simulink model "LKAS_AutoSave_20200911_1102"  (R2018b)
settings: Solver=FixedStepDiscrete  StartTime=0.0  StopTime=10.0  FixedStep=0.01  RelTol=1e-3
InitFcn:
  | tmpVer = ver('MATLAB');
  | tmpVer = str2num(tmpVer.Version);
  | % -------------------------------------------------------------------
  | %  MATLAB file generated by Simulink.saveVars on 21-Nov-2019 10:06:14
  | %  MATLAB version: 7.13.0.564 (R2011b)
  | % -------------------------------------------------------------------
  | 
  | 
  | SInt16 = Simulink.AliasType;
  | SInt16.Description = 'Num';
  | if (tmpVer > 7.11)
  | 	SInt16.DataScope = 'Auto';
  | end
  | SInt16.HeaderFile = 'Rte_Type.h';
  | SInt16.BaseType = 'int16';
  | 
  | SInt32 = Simulink.AliasType;
  | SInt32.Description = 'Num';
  | if (tmpVer > 7.11)
  | 	SInt32.DataScope = 'Auto';
  | end
  | SInt32.HeaderFile = 'Rte_Type.h';
  | SInt32.BaseType = 'int32';
  | 
  | SInt8 = Simulink.AliasType;
  | SInt8.Description = 'Num';
  | if (tmpVer > 7.11)
  | 	SInt8.DataScope = 'Auto';
  | end
  | SInt8.HeaderFile = 'Rte_Type.h';
  | SInt8.BaseType = 'int8';
  | 
  | T_A_m2_1024_1_u32 = Simulink.NumericType;
  | T_A_m2_1024_1_u32.Description = 'm2 (square meters  (m2))';
  | if (tmpVer > 7.11)
  | 	T_A_m2_1024_1_u32.DataScope = 'Auto';
  | end
  | T_A_m2_1024_1_u32.HeaderFile = 'Rte_Type.h';
  | T_A_m2_1024_1_u32.DataTypeMode = 'Fixed-point: slope and bias scaling';
  | T_A_m2_1024_1_u32.SignednessBool = false;
  | T_A_m2_1024_1_u32.WordLength = 32;
  | T_A_m2_1024_1_u32.FixedExponent = -10;
  | T_A_m2_1024_1_u32.SlopeAdjustmentFactor = 1;
  | T_A_m2_1024_1_u32.Bias = 0;
  | T_A_m2_1024_1_u32.DataTypeOverride = 'Inherit';
  | T_A_m2_1024_1_u32.IsAlias = true;
  | 
  | T_A_m2_65536_1_u16 = Simulink.NumericType;
  | T_A_m2_65536_1_u16.Description = 'm2 (square meters  (m2))';
  | if (tmpVer > 7.11)
  | 	T_A_m2_65536_1_u16.DataScope = 'Auto';
  | end
  | T_A_m2_65536_1_u16.HeaderFile = 'Rte_Type.h';
  | T_A_m2_65536_1_u16.DataTypeMode = 'Fixed-point: slope and bias scaling';
  | T_A_m2_65536_1_u16.SignednessBool = false;
  | T_A_m2_65536_1_u16.WordLength = 16;
  | T_A_m2_65536_1_u16.FixedExponent = -16;
  | T_A_m2_65536_1_u16.SlopeAdjustmentFactor = 1;
  | T_A_m2_65536_1_u16.Bias = 0;
  | T_A_m2_65536_1_u16.DataTypeOverride = 'Inherit';
  | ... (+4598 lines)
StopFcn:
  | clear  T_A_m2_1024_1_u32 T_A_m2_65536_1_u16 T_A_m2_Float32 T_A_mm2_10_1_u16 T_A_mm2_4_1_s16 T_A_mm2_Float32 T_Cnt_Num_10_1_u32 T_Cnt_Num_1_1_s16 T_Cnt_Num_1_1_s32 T_Cnt_Num_1_1_s8 T_Cnt_Num_1_1_u16 T_Cnt_Num_1_1_u32 T_Cnt_Num_1_1_u8 T_E_J_1_1_s32 T_E_J_Float32 T_E_kJ_128_1_s32 T_E_kJ_Float32 T_E_kwh_10_1_u16 T_E_kwh_Float32 T_Epl_kwhpkm_100_1_u16 T_Epl_kwhpkm_Float32 T_F_N_1_1_s16 T_F_N_Float32 T_I_A_1000_1_u16 T_I_A_1048576_1_s32 T_I_A_2048_1_s16 T_I_A_32_1_s16 T_I_A_Float32 T_I_mA_1_1_s16 T_I_mA_32768_128_s16 T_I_mA_Float32 T_J_kgpm2_128_1_u16 T_J_kgpm2_Float32 T_K_NA_1000_1_s16 T_K_NA_100_1_s16 T_K_NA_100_1_u16 T_K_NA_1024_1_s16 T_K_NA_1024_1_u16 T_K_NA_128_1_s16 T_K_NA_128_1_u16 T_K_NA_128_1_u8 T_K_NA_16777216_1_u32 T_K_NA_16_1_s16 T_K_NA_16_1_u16 T_K_NA_16_1_u8 T_K_NA_1_16_u16 T_K_NA_1_1_s16 T_K_NA_1_1_u16 T_K_NA_1_1_u8 T_K_NA_32768_1_s16 T_K_NA_32768_1_u16 T_K_NA_32_1_s8 T_K_NA_4096_1_u16 T_K_NA_4194304_1_s32 T_K_NA_4194304_1_u16 T_K_NA_65536_1_s32 T_K_NA_65536_1_u16 T_K_NA_8192_1_s16 T_K_NA_8_1_s16 T_K_NA_Float32 T_M_Nm_16_1_s16 T_M_Nm_1_1_s16 T_M_Nm_32768_1_s16 T_M_Nm_32_1_s16 T_M_Nm_4_1_s16 T_M_Nm_512_1_s16 T_M_Nm_Float32 T_P_W_1_4_s16 T_P_W_1_8_s16 T_P_W_Float32 T_P_kW_128_1_s16 T_P_kW_1_8_s16 T_P_kW_8_1_s32 T_P_kW_Float32 T_Pct_pct_1024_1_s32 T_Pct_pct_1024_1_u32 T_Pct_pct_10_1_s16 T_Pct_pct_10_1_u32 T_Pct_pct_128_100_s8 T_Pct_pct_1_1_s16 T_Pct_pct_1_4_u8 T_Pct_pct_255_100_u16 T_Pct_pct_255_100_u8 T_Pct_pct_256_1_s16 T_Pct_pct_256_1_u16 T_Pct_pct_65535_100_u16 T_Pct_pct_Float32 T_R_ohm_1024_1_s16 T_R_ohm_32_1_s16 T_R_ohm_Float32 T_TK_K_16_1_s16 T_TK_K_Float32 T_T_degC_10_400_1_u16 T_T_degC_16_1_s16 T_T_degC_1_40_1_u8 T_T_degC_2_80_1_u8 T_T_degC_Float32 T_U_V_1000_1_u16 T_U_V_10_1_u8 T_U_V_200_1_u8 T_U_V_32_1_s16 T_U_V_4096_1_s16 T_U_V_512_1_s16 T_U_V_65535_8_u16 T_U_V_8192_1_u16 T_U_V_Float32 T_U_mV_1_1_s16 T_U_mV_256_20_u16 T_U_mV_Float32 T_V_l_256_1_s16 T_V_l_4096_1_s16 T_V_l_64_1_s16 T_V_l_65535_100_u16 T_V_l_Float32 T_V_ml_128_1_s16 T_V_ml_1_1_s16 T_V_ml_32768_1_s16 T_V_ml_Float32 T_V_ul_32_1_u16 T_V_ul_Float32 T_Vpl_clpkm_512_1_u16 T_Vpl_clpkm_Float32 T_a_kphps_16_1_s16 T_a_kphps_Float32 T_a_mps2_128_1_s16 T_a_mps2_Float32 T_c_MJpkg_256_1_s16 T_c_MJpkg_Float32 T_c_kJpgpK_1024_1_s16 T_c_kJpgpK_Float32 T_c_kJpkgpK_128_1_u16 T_c_kJpkgpK_Float32 T_chrg_Ah_1_1_s16 T_chrg_Ah_1_1_u16 T_chrg_Ah_1_1_u8 T_chrg_Ah_256_1_u16 T_chrg_Ah_4194304_1_s32 T_chrg_Ah_512_1_u16 T_chrg_Ah_8_1_u16 T_chrg_Ah_Float32 T_cmp_NA_100_1_s16 T_cmp_NA_128_1_s16 T_cmp_NA_16_1_s16 T_cmp_NA_32768_1_u16 T_cmp_NA_Float32 T_d2n_rpmps2_4_1_s16 T_d2n_rpmps2_Float32 T_dPct_pctps_16_1_s16 T_dPct_pctps_256_1_s16 T_dPct_pctps_Float32 T_dT_degCps_128_1_s16 T_dT_degCps_Float32 T_dV_lph_1_1_s16 T_dV_lph_Float32 T_dV_lpm_128_1_s16 T_dV_lpm_32_1_s16 T_dV_lpm_Float32 T_dV_lps_1024_1_u16 T_dV_lps_4_1_u16 T_dV_lps_Float32 T_dV_mlps_1024_1_s16 T_dV_mlps_Float32 T_d_BitField16 T_dm_gps_128_1_s16 T_dm_gps_128_1_u16 T_dm_gps_256_1_u16 T_dm_gps_Float32 T_dm_mgps_1_1_s16 T_dm_mgps_Float32 T_dn_rpmps_1_1_s16 T_dn_rpmps_2_1_s16 T_dn_rpmps_Float32 T_dp_Paps_1_1_s16 T_dp_Paps_Float32 T_dp_kPaps_1_1_s16 T_dp_kPaps_8_1_s16 T_dp_kPaps_Float32 T_dphi_degps_128_1_s16 T_dphi_degps_8_1_s16 T_dphi_degps_Float32 T_dr_ps_256_1_s16 T_dr_ps_Float32 T_drho_mgplps_1_2_s16 T_drho_mgplps_Float32 T_e_NA_1_1_u8 T_f_Hz_1_1_u16 T_f_Hz_1_1_u32 T_f_Hz_64_1_u16 T_f_Hz_8_1_s16 T_f_Hz_Float32 T_g_BitField32 T_l_km_16_1_s16 T_l_km_1_1_u16 T_l_km_1_1_u32 T_l_km_Float32 T_l_m_1024_1_s16 T_l_m_16_1_s16 T_l_m_1_1_u32 T_l_m_Float32 T_l_mm_16_1_s16 T_l_mm_1_1_u16 T_l_mm_4096_1_s16 T_l_mm_4_1_u8 T_l_mm_64_1_s16 T_l_mm_Float32 T_m_g_1_1_s16 T_m_g_2048_1_s16 T_m_g_32_1_u16 T_m_g_Float32 T_m_kg_1024_1_s16 T_m_kg_1_1_s16 T_m_kg_1_1_u32 T_m_kg_Float32 T_m_mg_128_1_s16 T_m_mg_32_1_s16 T_m_mg_Float32 T_n_rpm_1_1_s16 T_n_rpm_1_25_u8 T_n_rpm_256_50_u16 T_n_rpm_2_25_u8 T_n_rpm_4_1_u16 T_n_rpm_Float32 T_p_MPa_64_1_s16 T_p_MPa_Float32 T_p_Pa_1_1_s16 T_p_Pa_Float32 T_p_kPa_1_10_u16 T_p_kPa_1_1_s16 T_p_kPa_1_1_u8 T_p_kPa_256_1_u16 T_p_kPa_32_1_u16 T_p_kPa_64_1_s16 T_p_kPa_Float32 T_phi_deg_100_1_s16 T_phi_deg_1024_1_s16 T_phi_deg_128_1_s16 T_phi_deg_1_1_u8 T_phi_deg_256_1_s16 T_phi_deg_2_1_s8 T_phi_deg_32_1_s16 T_phi_deg_512_6_s32 T_phi_deg_Float32 T_phi_rad_2048_1_s16 T_phi_rad_Float32 T_r_NA_1024_1_s16 T_r_NA_1024_1_u16 T_r_NA_16384_1_s16 T_r_NA_16_1_s16 T_r_NA_256_1_s8 T_r_NA_256_1_u16 T_r_NA_32768_1_u16 T_r_NA_32_1_u16 T_r_NA_4096_1_s16 T_r_NA_65535_2_u16 T_r_NA_8192_1_u16 T_r_NA_Float32 T_rho_gpl_8192_1_s16 T_rho_gpl_Float32 T_rho_kgpm3_16_1_s16 T_rho_kgpm3_Float32 T_rho_mgpl_1_1_s16 T_rho_mgpl_64_1_s16 T_rho_mgpl_Float32 T_t_hour_1_1_s16 T_t_hour_Float32 T_t_m_1_1_u16 T_t_m_Float32 T_t_ms_1_1_s16 T_t_ms_1_1_u16 T_t_ms_1_1_u32 T_t_ms_4096_1_s16 T_t_ms_64_1_s16 T_t_ms_Float32 T_t_s_1000_1_s16 T_t_s_100_1_s16 T_t_s_10_1_s16 T_t_s_10_1_u16 T_t_s_1_1_s16 T_t_s_1_1_u16 T_t_s_1_1_u32 T_t_s_Float32 T_t_us_10_1_u32 T_t_us_1_1_s16 T_t_us_1_1_u32 T_t_us_1_4_u16 T_t_us_Float32 T_v_kph_1_1_u8 T_v_kph_64_1_s16 T_v_kph_64_1_u16 T_v_kph_Float32 T_v_mps_256_1_s16 T_v_mps_Float32 T_w_radps_32_1_s16 T_w_radps_Float32 T_y_BitField8 T_y_BitFieldDiagProgress T_y_BitFieldDiagStatus T_y_NA_1_1_u8 SInt16 SInt32 SInt8 T_BOOLEAN UInt16 UInt32 UInt8 s16 s32 s8 u16 u32 u8
model workspace (MAT data in the model file):
  MCOS : class17 (value not decoded)
  MCOS : class17 (value not decoded)
  MCOS : class17 (value not decoded)
  MCOS : class17 (value not decoded)
  MCOS : class17 (value not decoded)
  MCOS : class17 (value not decoded)
  MCOS : class17 (value not decoded)
  MCOS : class17 (value not decoded)
  MCOS : class17 (value not decoded)
  MCOS : class17 (value not decoded)
  MCOS : class17 (value not decoded)
  MCOS : class17 (value not decoded)
  MCOS : class17 (value not decoded)
  MCOS : class17 (value not decoded)
  MCOS : class17 (value not decoded)
  MCOS : class17 (value not decoded)
  MCOS : class17 (value not decoded)
  MCOS : class17 (value not decoded)
  MCOS : class17 (value not decoded)
  MCOS : class17 (value not decoded)
  MCOS : class17 (value not decoded)
  MCOS : class17 (value not decoded)
  MCOS : class17 (value not decoded)
  MCOS : class17 (value not decoded)
  MCOS : class17 (value not decoded)
  MCOS : class17 (value not decoded)
  MCOS : class17 (value not decoded)
  MCOS : class17 (value not decoded)
  MCOS : class17 (value not decoded)
  MCOS : class17 (value not decoded)
  MCOS : class17 (value not decoded)
  MCOS : class17 (value not decoded)
  MCOS : class17 (value not decoded)
  MCOS : class17 (value not decoded)
  MCOS : class17 (value not decoded)
  MCOS : class17 (value not decoded)
  MCOS : class17 (value not decoded)
  MCOS : class17 (value not decoded)
  MCOS : class17 (value not decoded)
  MCOS : class17 (value not decoded)
  MCOS : class17 (value not decoded)
  MCOS : class17 (value not decoded)
  MCOS : class17 (value not decoded)
  MCOS : class17 (value not decoded)
  MCOS : class17 (value not decoded)
  MCOS : class17 (value not decoded)
  MCOS : class17 (value not decoded)
  MCOS : class17 (value not decoded)
  MCOS : class17 (value not decoded)
  MCOS : class17 (value not decoded)
  MCOS : class17 (value not decoded)
  MCOS : class17 (value not decoded)
  MCOS : class17 (value not decoded)
  MCOS : class17 (value not decoded)
  MCOS : class17 (value not decoded)
  MCOS : class17 (value not decoded)
  MCOS : class17 (value not decoded)
  MCOS : class17 (value not decoded)
  MCOS : class17 (value not decoded)
  MCOS : class17 (value not decoded)
  MCOS : class17 (value not decoded)
  MCOS : class17 (value not decoded)
  MCOS : class17 (value not decoded)
  MCOS : class17 (value not decoded)
  MCOS : class17 (value not decoded)
  MCOS : class17 (value not decoded)
  MCOS : class17 (value not decoded)
  MCOS : class17 (value not decoded)
  MCOS : class17 (value not decoded)
  MCOS : class17 (value not decoded)
  MCOS : class17 (value not decoded)
  MCOS : class17 (value not decoded)
  MCOS : class17 (value not decoded)
  MCOS : class17 (value not decoded)
  MCOS : class17 (value not decoded)
  MCOS : class17 (value not decoded)
  MCOS : class17 (value not decoded)
  MCOS : class17 (value not decoded)
  MCOS : class17 (value not decoded)
  MCOS : class17 (value not decoded)
  MCOS : class17 (value not decoded)
  MCOS : class17 (value not decoded)
  MCOS : class17 (value not decoded)
  MCOS : class17 (value not decoded)
  MCOS : class17 (value not decoded)
  MCOS : class17 (value not decoded)
  MCOS : class17 (value not decoded)
  MCOS : class17 (value not decoded)
  MCOS : class17 (value not decoded)
undefined symbols (not defined in the file): LKA_CarWidth, LKA_SampleTime, LKA_StrRatio_C, LKA_Veh2CamL_C, LKA_Veh2CamW_C, LKA_WhlBaseL_C, LL_CompSWA_C, LL_CrvtPrvwT_C, LL_DesDvt_C, LL_DvtComp_C, LL_DvtPrvwT_C, LL_DvtSpdDet_vDvtSpdMin_C, LL_HdAgExT_C, LL_HdAgPrvwT_C, LL_LAccMax_C, LL_LAccRMax_C, LL_LDW_EarliestWarnLine_C, LL_LDW_LatestWarnLine_C, LL_LDWS_SUPPRESS_HEADING, LL_LFClb_TFC_DiffCtlBalance, LL_LFClb_TFC_DiffCtrlMaxSWA, LL_LFClb_TFC_DiffCtrlRatio, LL_LFClb_TFC_facmGainLutGain1_C, LL_LFClb_TFC_facmGainLutGain2_C, LL_LFClb_TFC_facmIntegRatio, LL_LFClb_TFC_facmKlat_C, LL_LFClb_TFC_FfCtlRatio_C, LL_LFClb_TFC_phiIntegCtlMaxSWA_C, LL_LFClb_TFC_tiKlatPrvwT_C, LL_LFClb_TFC_vGainLutVehSpdLwr_C, LL_LFClb_TFC_vGainLutVehSpdUpr_C, LL_LKA_EarliestWarnLine_C, LL_LKA_LatestWarnLine_C, LL_LKAExPrcs_ExitC0Dvt, LL_LKAExPrcs_ExitC0Swt, LL_LKAExPrcs_tiExitTime1, LL_LKAExPrcs_tiExitTime2, LL_LKAExPrcs_tiExitTime3, LL_LKAS_OUT_OF_CONTROL_LAT_VEL, LL_LKAS_OUT_OF_CONTROL_TTLC, LL_LKASWASyn_M0, LL_LKASWASyn_M1, LL_LKASWASyn_M2, LL_LKASWASyn_M3K, LL_LKASWASyn_SWAaddMax, LL_LKASWASyn_T2, LL_LKASWASyn_tiTrqSwaRtTime, LL_LKASWASyn_tiTrqSwaTime, LL_LKASWASyn_TrqMax, LL_LKASWASyn_TrqSwaAddSwt, LL_LKASWASyn_TrqSwaRateDiff, LL_LSpdCompT_C, LL_lStpLngth_C, LL_MAX_DELAY_EPSSTAR_TIME, LL_MAX_DRIVER_TORQUE_DISABLE, LL_MAX_DRIVER_TORQUE_ENABLE, LL_MAX_LANE_WIDTH_DISABLE, LL_MAX_LANE_WIDTH_ENABLE, LL_MAX_LAT_ACC_DISABLE, LL_MAX_LAT_ACC_ENABLE ... (+29)
libraries: simulink x134, dspstat3 x3, simulink_extras x1
(part 18 of 19)

== matlab function LKAS_AutoSave_20200911_1102/LKAS/LL/Human Machine Interface (HMI)/HMI_Popup_Status ==
  data: HMI_Popup_Status output; stDACmode input; LKA_STATE input; HandsOff input; camera_common_fault input; Front_Camera_Blocked input; stFaultCSyn input
function HMI_Popup_Status = fcn(stDACmode,LKA_STATE,HandsOff,camera_common_fault,Front_Camera_Blocked,stFaultCSyn)
if stDACmode==2&&LKA_STATE==6 %车道保持辅助故障
    HMI_Popup_Status=uint8(6);
elseif stDACmode==2&&camera_common_fault==1&&Front_Camera_Blocked~=5  %车道保持辅助暂不可用
    HMI_Popup_Status=uint8(3);
elseif (stDACmode==2||stDACmode==1)&&(Front_Camera_Blocked==5)   %摄像头被遮挡
    HMI_Popup_Status=uint8(4);
elseif (stDACmode==2||stDACmode==1)&&HandsOff==1  %手握方向盘
    HMI_Popup_Status=uint8(2);    
elseif stDACmode==2&&(LKA_STATE==2)
    HMI_Popup_Status=uint8(1);
elseif stDACmode~=2&&stFaultCSyn==0
    HMI_Popup_Status=uint8(8);
elseif stFaultCSyn==0
    HMI_Popup_Status=uint8(7);
elseif stDACmode==2&&(LKA_STATE==0||LKA_STATE==1)
    HMI_Popup_Status=uint8(0);
else
    HMI_Popup_Status=uint8(0);
end

== matlab function LKAS_AutoSave_20200911_1102/LKAS/LL/Human Machine Interface (HMI)/Hands_off_warning ==
  data: Hands_off_warning output; HandsOff input
function Hands_off_warning = fcn(HandsOff)
Hands_off_warning = uint8(0);
if HandsOff==0
    Hands_off_warning= uint8(0);
elseif HandsOff==1
    Hands_off_warning= uint8(1);
else
    Hands_off_warning= uint8(0);
end

== matlab function LKAS_AutoSave_20200911_1102/LKAS/LL/Human Machine Interface (HMI)/LDW_Flag ==
  data: HMI_stDACmode input; HMI_LKA_STATE input; LDW_Flag output; HMI_LDWWarnInfo input
function LDW_Flag = fcn(HMI_stDACmode, HMI_LKA_STATE, HMI_LDWWarnInfo)
if HMI_stDACmode==1
    LDW_Flag = uint8(0);
    if HMI_LDWWarnInfo==1
        LDW_Flag=uint8(1);
    elseif HMI_LDWWarnInfo==2
        LDW_Flag=uint8(2);
    else
        LDW_Flag=uint8(0);
    end
elseif HMI_stDACmode==2
    LDW_Flag = uint8(0);
    if HMI_LDWWarnInfo==1 && HMI_LKA_STATE==4
        LDW_Flag=uint8(1);
    elseif HMI_LDWWarnInfo==2 && HMI_LKA_STATE==5
        LDW_Flag=uint8(2);
    else
        LDW_Flag=uint8(0);
    end    
else
    LDW_Flag=uint8(0);
end
end

== matlab function LKAS_AutoSave_20200911_1102/LKAS/LL/Human Machine Interface (HMI)/LDW_Status_Display ==
  data: stDACmode input; LDW_Status_Display output; LDW_STATE input
function LDW_Status_Display = fcn(stDACmode,LDW_STATE)
if (stDACmode==1)&&LDW_STATE~=6
    LDW_Status_Display=uint8(1);
elseif (stDACmode==1)&&LDW_STATE==6
    LDW_Status_Display=uint8(2);
else
    LDW_Status_Display=uint8(0);
end

== matlab function LKAS_AutoSave_20200911_1102/LKAS/LL/Human Machine Interface (HMI)/LKA_Status_Display ==
  data: stDACmode input; LKA_Status_Display output; LKA_STATE input
function LKA_Status_Display  = fcn(stDACmode,LKA_STATE)
LKA_Status_Display = single(0);
if stDACmode==2&&LKA_STATE~=6
    LKA_Status_Display=single(1);
elseif stDACmode==2&&LKA_STATE==6
    LKA_Status_Display=single(2);
else
    LKA_Status_Display=single(0);
end

== matlab function LKAS_AutoSave_20200911_1102/LKAS/LL/Human Machine Interface (HMI)/LKA_action_indication ==
  data: LKA_action_indication output; stDACmode input; LKA_STATE input
function LKA_action_indication = fcn(stDACmode,LKA_STATE)
if stDACmode==2&&LKA_STATE==2
    LKA_action_indication=uint8(1);
elseif stDACmode==2&&LKA_STATE==3
    LKA_action_indication=uint8(2);
elseif stDACmode==2&&(LKA_STATE==4||LKA_STATE==5)
    LKA_action_indication=uint8(3);
else
    LKA_action_indication=uint8(0);
end

== matlab function LKAS_AutoSave_20200911_1102/LKAS/LL/Human Machine Interface (HMI)/Vehicle_Lane_Display ==
  data: stDACmode input; Vehicle_Lane_Display output; LKA_STATE input; LDW_STATE input; R0_Quality input; L0_Quality input
function Vehicle_Lane_Display = fcn(stDACmode,LKA_STATE,LDW_STATE,R0_Quality,L0_Quality)
if stDACmode==1
    if LDW_STATE==3 && L0_Quality==3 && R0_Quality~=3
        Vehicle_Lane_Display=uint8(3);
    elseif LDW_STATE==3 && L0_Quality~=3 && R0_Quality==3
        Vehicle_Lane_Display=uint8(4);
    elseif LDW_STATE==3 && L0_Quality==3 && R0_Quality==3
        Vehicle_Lane_Display=uint8(5);
    elseif LDW_STATE==4 && L0_Quality==3 && R0_Quality~=3
        Vehicle_Lane_Display=uint8(6);
    elseif LDW_STATE==5 && L0_Quality~=3 && R0_Quality==3
        Vehicle_Lane_Display=uint8(7);
    elseif LDW_STATE==4 && L0_Quality==3 && R0_Quality==3
        Vehicle_Lane_Display=uint8(8);
    elseif LDW_STATE==5 && L0_Quality==3 && R0_Quality==3
        Vehicle_Lane_Display=uint8(9);
    else
        Vehicle_Lane_Display=uint8(1);
    end
elseif stDACmode==2
    if LKA_STATE==3 && L0_Quality==3 && R0_Quality~=3
        Vehicle_Lane_Display=uint8(3);
    elseif LKA_STATE==3 && L0_Quality~=3 && R0_Quality==3
        Vehicle_Lane_Display=uint8(4);
    elseif LKA_STATE==3 && L0_Quality==3 && R0_Quality==3
        Vehicle_Lane_Display=uint8(5);
    elseif LKA_STATE==4 && L0_Quality==3 && R0_Quality~=3
        Vehicle_Lane_Display=uint8(6);
    elseif LKA_STATE==5 && L0_Quality~=3 && R0_Quality==3
        Vehicle_Lane_Display=uint8(7);
    elseif LKA_STATE==4 && L0_Quality==3 && R0_Quality==3
        Vehicle_Lane_Display=uint8(8);
    elseif LKA_STATE==5 && L0_Quality==3 && R0_Quality==3
        Vehicle_Lane_Display=uint8(9);
    else
        Vehicle_Lane_Display=uint8(1);
    end
else
    Vehicle_Lane_Display=uint8(0);
end

== stateflow chart LKAS_AutoSave_20200911_1102/LKAS/LL/LL Inputs Mapping/bsLaneInfo/LanesReconstruct /LaneReconstructSM ==
  state NoLaneLost
    en:LaneRSM_stRoadFlg=uint8(1);
    LaneRSM_stLftFlg=uint8(1);
    LaneRSM_stRgtFlg=uint8(1);
  state RightLost
    en:LaneRSM_stRoadFlg=uint8(0);
    LaneRSM_stLftFlg=uint8(1);
    LaneRSM_stRgtFlg=uint8(0);
  state LeftLost
    en:LaneRSM_stRoadFlg=uint8(0);
    LaneRSM_stLftFlg=uint8(0);
    LaneRSM_stRgtFlg=uint8(1);
  state DoubleLost
  LeftLost -> RightLost [order 2] : [LaneRSM_stL0Ql==3&&LaneRSM_stR0Ql<3]
  (default) -> NoLaneLost
  NoLaneLost -> LeftLost [order 1] : [LaneRSM_stL0Ql<3&&LaneRSM_stR0Ql==3]
  NoLaneLost -> RightLost [order 2] : [LaneRSM_stL0Ql==3&&LaneRSM_stR0Ql<3]
  LeftLost -> NoLaneLost [order 1] : [LaneRSM_stL0Ql==3&&LaneRSM_stR0Ql==3]
  RightLost -> NoLaneLost [order 1] : [LaneRSM_stL0Ql==3&&LaneRSM_stR0Ql==3]
  NoLaneLost -> DoubleLost [order 3] : [LaneRSM_stL0Ql<3&&LaneRSM_stR0Ql<3]{LaneRSM_stRoadFlg=uint8(0);}
  DoubleLost -> NoLaneLost [order 1] : [LaneRSM_stL0Ql==3&&LaneRSM_stR0Ql==3]
  RightLost -> LeftLost [order 2] : [LaneRSM_stL0Ql<3&&LaneRSM_stR0Ql==3]
  RightLost -> DoubleLost [order 3] : [LaneRSM_stL0Ql<3]
  DoubleLost -> RightLost [order 2] : [LaneRSM_stL0Ql==3&&LaneRSM_stR0Ql<3]
  LeftLost -> DoubleLost [order 3] : [LaneRSM_stR0Ql<3]
  DoubleLost -> LeftLost [order 3] : [LaneRSM_stL0Ql<3&&LaneRSM_stR0Ql==3]
  data: LaneRSM_stL0Ql input uint8; LaneRSM_stR0Ql input uint8; LaneRSM_stRoadFlg output uint8; LaneRSM_stLftFlg output uint8; LaneRSM_stRgtFlg output uint8

== matlab function LKAS_AutoSave_20200911_1102/LKAS/LL/LL Inputs Mapping/bsLaneInfo/LanesReconstruct /RoadSide Offset/get_roadside_offset ==
  data: cur input; offset output; lanewidth input
function offset = fcn(cur,lanewidth)
lanewidth=min(single(4),lanewidth);
cur=min(single(0.004),cur);
offset=(cur/single(0.004)+single(1))*single(0.2)*(lanewidth-single(2)); %% 车道线宽4米，路沿可以偏置0.4，宽3m，路沿可以偏置，0.2m
offset=min(single(0.5),offset);
end

== matlab function LKAS_AutoSave_20200911_1102/LKAS/LL/LLOn/LDW/LDWWarnInfo ==
  data: LDW_stLDWActvFlg input; LDWWarnInfo output; LDW_stHdAgDetFlg input
function LDWWarnInfo = fcn(LDW_stLDWActvFlg,LDW_stHdAgDetFlg)
if LDW_stLDWActvFlg==1&&LDW_stHdAgDetFlg==0
    LDWWarnInfo=uint8(1);
elseif LDW_stLDWActvFlg==2&&LDW_stHdAgDetFlg==0
    LDWWarnInfo=uint8(2);
else
    LDWWarnInfo=uint8(0);
end

== matlab function LKAS_AutoSave_20200911_1102/LKAS/LL/LLOn/LKA/Driver Torque Addition (DTA)/Subsystem/DriverSwaTrqAdd ==
  data: spd input; Swaadd output single; trq input; l0c0 input; r0c0 input; swaaddmax input; trqmax input
function Swaadd = fcn(spd,trq,l0c0,r0c0,swaaddmax,trqmax)
Swaadd=single(0);
spd=max(min(spd,single(120)),single(60));%对输入车速进行限制在60~120km/h
swaaddmax=(single(180)-spd)/single(120)*swaaddmax;%根据当前车速限制方向盘叠加最大值=(1~0.5)*spdaddmax
l0c0=abs(l0c0);
r0c0=abs(r0c0);
lanewidth=max(min(l0c0+r0c0,single(5.4)),single(2.5));
if lanewidth>single(2.5) && lanewidth<single(5.4)
    leftlane=l0c0/lanewidth;
    rightlane=r0c0/lanewidth;
else
    leftlane=single(0.5);
    rightlane=single(0.5);
end
leftswamax=single(2)*swaaddmax*leftlane;
rightswamax=single(2)*swaaddmax*rightlane;
if trq>=0
    Swaadd=trq/trqmax*leftswamax;
else
    Swaadd=trq/trqmax*rightswamax;
end

== matlab function LKAS_AutoSave_20200911_1102/LKAS/LL/LLOn/LKA/Driver Torque Addition (DTA)/Subsystem1/MATLAB Function ==
  data: M0 input; M output; M1 input; M2 input; T1 input; T2 input; T input
function M = fcn(M0,M1,M2,T1,T2,T)
    if T<T1
        M = M0+(M1-M0)/T1*T;
    elseif T>=T1 && T<=(T1+T2)
        M = (M2-M1)/(T2)*(T-T1)+M1;
    else
        M = M2;
    end
end

== matlab function LKAS_AutoSave_20200911_1102/LKAS/LL/LLOn/LKA/LKA Motion Planning (LKAMP) /LKA Motion Planning Calculation (LKAMPCal)/MATLAB Function ==
  data: K1K2Det_stLDDir input; K1K2Det_dphi1PhSWAGrad output; K1K2Det_tiTTLC0 input; K1K2Det_vVehSpd input; K1K2Det_phiIniSWA input; K1K2Det_phiPrvwHdAgIni input; K1K2Det_phiTTLCHdAgIni input; K1K2Det_phi1PhDesHdAgIni input; K1K2Det_phi2PhDesHdAg input; K1K2Det_l1PhDvtIni input; K1K2Det_dphiSWARMax input; K1K2Det_crPrvwTTLCCrvt input; K1K2Det_bsTDivInfo_ModeFlg input; K1K2Det_bsTDivInfo_Mode1Num input; K1K2Det_bsTDivInfo_Mode2Num input; K1K2Det_bsTDivInfo_Ph2DvtEnd input; K1K2Det_bsTDivInfo_Ph2SWAIni input; K1K2Det_lDesDvt input; K1K2Det_lStpLngth input; K1K2Det_bsSysCfg_SY_WhlBase_SY input; K1K2Det_bsSysCfg_SY_StRatio_SY input; K1K2Det_bsSysCfg_SY_StbFacm_SY input; K1K2Det_dphi2PhSWAGrad1 output; K1K2Det_dphi2PhSWAGrad2 output; K1K2Det_phi2PhSWAIni output; K1K2Det_stReplFlag output; K1K2Det_dphi1PhHdAgIni output; K1K2Det_bsTDivInfoOut_ModeFlg output; K1K2Det_bsTDivInfoOut_Mode1Num output; K1K2Det_bsTDivInfoOut_Mode2Num output; K1K2Det_bsTDivInfoOut_Ph2DvtEnd output; K1K2Det_bsTDivInfoOut_Ph2SWAIni output
  function [K1K2Det_dphi1PhSWAGrad,...
            K1K2Det_dphi2PhSWAGrad1,...
            K1K2Det_dphi2PhSWAGrad2,...
            K1K2Det_phi2PhSWAIni,...
            K1K2Det_stReplFlag,...
            K1K2Det_dphi1PhHdAgIni,...
            K1K2Det_bsTDivInfoOut_ModeFlg,...
            K1K2Det_bsTDivInfoOut_Mode1Num,...
            K1K2Det_bsTDivInfoOut_Mode2Num,...
            K1K2Det_bsTDivInfoOut_Ph2DvtEnd,...
            K1K2Det_bsTDivInfoOut_Ph2SWAIni]= K1K2Det(K1K2Det_stLDDir,... 
                                          K1K2Det_tiTTLC0,...                                        
                                          K1K2Det_vVehSpd,...
                                          K1K2Det_phiIniSWA,...
                                          K1K2Det_phiPrvwHdAgIni,... 
                                          K1K2Det_phiTTLCHdAgIni,... 
                                          K1K2Det_phi1PhDesHdAgIni,... 
                                          K1K2Det_phi2PhDesHdAg,...
                                          K1K2Det_l1PhDvtIni,...
                                          K1K2Det_dphiSWARMax,...
                                          K1K2Det_crPrvwTTLCCrvt,...
                                          K1K2Det_bsTDivInfo_ModeFlg,...
                                          K1K2Det_bsTDivInfo_Mode1Num,...
                                          K1K2Det_bsTDivInfo_Mode2Num,...
                                          K1K2Det_bsTDivInfo_Ph2DvtEnd,...
                                          K1K2Det_bsTDivInfo_Ph2SWAIni,...
                                          K1K2Det_lDesDvt,...
                                          K1K2Det_lStpLngth,...
                                          K1K2Det_bsSysCfg_SY_WhlBase_SY,...
                                          K1K2Det_bsSysCfg_SY_StRatio_SY,...
                                          K1K2Det_bsSysCfg_SY_StbFacm_SY)...
                                       
% *************************************************************************
% 输入量：
%   K1K2Det_stLDDir : 车辆的车道偏离的方向。1代表车辆向右侧车道线偏出，-1代表车辆
%                       向左侧车道线偏出。单位：-
%   K1K2Det_tiTTLC0 : 进入一区时的TTLC，单位：s
%   K1K2Det_vVehSpd : 车速，单位：Km/h
%   K1K2Det_phiIniSWA : 初始转向盘转角，单位：deg
%   K1K2Det_phi1PhDesHdAgChg : 一区期望航向角变化量,单位：radian
%   K1K2Det_phi2PhDesHdAg : 二区结束时的期望航向角，单位：radian
%   K1K2Det_l1PhDvtIni : 进入一区时的偏移量初值，单位：m
%   K1K2Det_lDesDvt : 二区结束时的期望偏移量的绝对值，单位：m
% 标定量：
%   WhlBase_SY : 车辆轴距，单位：m
%   StRatio_SY : 转向传动比，单位：-
%   StbFacm_SY : 稳定性因数，单位：-
% 输出量：
%   K1K2Det_dphi1PhSWAGrad : 一区转向盘转角变化率，单位：deg/s
%   K1K2Det_dphi2PhSWAGrad1 : 二区转向盘转角变化率1，单位：deg/s
%   K1K2Det_dphi2PhSWAGrad2 ：二区转向盘转角变化率2，单位：deg/s
%   K1K2Det_phi2PhSWAIni : 二区转向盘转角初始值，单位：deg
%   K1K2Det_stReplFlag : 重新规划标志，单位：-
%**************************************************************************
    LDDir = K1K2Det_stLDDir;
    D1_Ini = K1K2Det_l1PhDvtIni;
    D2_des = K1K2Det_lDesDvt;
    DelteSW0 = K1K2Det_phiIniSWA*(pi/180);
    PrvwHdAg = K1K2Det_phiPrvwHdAgIni;
    TTLCHdAg = K1K2Det_phiTTLCHdAgIni;
    Delte_Psi2 = K1K2Det_phi2PhDesHdAg;
    Delte_Psi1Ini = K1K2Det_phi1PhDesHdAgIni;
    TTLC = single(K1K2Det_tiTTLC0);
    TTLCCrvt = K1K2Det_crPrvwTTLCCrvt;
    L = K1K2Det_bsSysCfg_SY_WhlBase_SY;
    i = K1K2Det_bsSysCfg_SY_StRatio_SY;
    K = K1K2Det_bsSysCfg_SY_StbFacm_SY;
    u = K1K2Det_vVehSpd/3.6;
    Kw=u/(L*(1+K*u*u)*i);
%     DelteSW1 = single(0);
    K1K2Det_stReplFlag = single(0);
    StpLngth = K1K2Det_lStpLngth*(pi/180);
    ModeFlg = K1K2Det_bsTDivInfo_ModeFlg;
    Mode1Num = K1K2Det_bsTDivInfo_Mode1Num;
    Mode2Num = K1K2Det_bsTDivInfo_Mode2Num;
    D2_End =  K1K2Det_bsTDivInfo_Ph2DvtEnd;
    DelteSW1 = K1K2Det_bsTDivInfo_Ph2SWAIni;
    K1 = single(0);
    K2_1 = single(0);
    K2_2 = single(0);
    KMax = K1K2Det_dphiSWARMax;
%**************************************************************************
%
% if (LDDir*PrvwHdAg < LDDir*TTLCHdAg)
%     Delte_Psi1 = PrvwHdAg;
% else
%     Delte_Psi1 = TTLCHdAg;
% end
Delte_Psi1 = PrvwHdAg;
if (ModeFlg == 0)
    [K1,K2_1,K2_2,D2_End,DelteSW1]= func1(Delte_Psi1,TTLC,Kw,DelteSW0,Delte_Psi2,u,D1_Ini,Delte_Psi1Ini);
end
if(0< D2_End*LDDir && D2_End*LDDir <= D2_des && ModeFlg == 0)
    
    K1K2Det_stReplFlag = single(0);
       
elseif(D2_End*LDDir > D2_des || ModeFlg ~= 0 )
    
    K1K2Det_stReplFlag = single(1);
    
    for a = 1:8

        if (D2_End*LDDir>D2_des && ModeFlg==0)
            ModeFlg = uint16(1);
        end
        if (D2_End*LDDir>D2_des && ModeFlg==1)
           DelteSW1 =  LDDir*StpLngth+DelteSW1;
           Mode1Num = Mode1Num+1;
        end
        if (D2_End*LDDir <= D2_des && ModeFlg==1)
            ModeFlg = uint16(2);
        end
        if (D2_End*LDDir<D2_des && ModeFlg==2)
           DelteSW1 =  DelteSW1-LDDir*StpLngth*((1/2)^(Mode2Num+1)); 
           Mode2Num = Mode2Num+1;
        end
        if (D2_End*LDDir>=D2_des && ModeFlg==2)
           DelteSW1 =  DelteSW1+LDDir*StpLngth*((1/2)^(Mode2Num+1)); 
           Mode2Num = Mode2Num+1;
        end
       [T1,T2,D2_End] = func3(Delte_Psi1Ini,Delte_Psi2,DelteSW1,KMax,Delte_Psi1,...
                                DelteSW0,u,Kw,LDDir);
    end
    K1 = (DelteSW1-DelteSW0)/T1;
    K2_1 = (0-DelteSW1)/T2;
    K2_2 = K2_1;
end %

%   K1K2Det_phi2PhSWAIni : 二区转向盘转角初始值，单位：deg
    K1K2Det_phi2PhSWAIni = DelteSW1*(180/pi);          
%   K1K2Det_dphi1PhSWAGrad : 一区转向盘转角变化率，单位：deg/s
    K1K2Det_dphi1PhSWAGrad = K1*(180/pi);
%   K1K2Det_dphi2PhSWAGrad1 : 二区转向盘转角变化率1，单位：deg/s
    K1K2Det_dphi2PhSWAGrad1 = K2_1*(180/pi);
%   K1K2Det_dphi2PhSWAGrad2 ：二区转向盘转角变化率2，单位：deg/s
    K1K2Det_dphi2PhSWAGrad2 = K2_2*(180/pi);
%
    K1K2Det_dphi1PhHdAgIni = Delte_Psi1;
%
    K1K2Det_bsTDivInfoOut_ModeFlg = ModeFlg;
    K1K2Det_bsTDivInfoOut_Mode1Num = Mode1Num;
    K1K2Det_bsTDivInfoOut_Mode2Num = Mode2Num;
    K1K2Det_bsTDivInfoOut_Ph2DvtEnd = D2_End;   
    K1K2Det_bsTDivInfoOut_Ph2SWAIni = DelteSW1;

end % end of function K1K2Det
%
%*****************************************
% 1、调用func1，输出二区结束时的偏移量计算值偏移量D2_0;
%    
% 2、若D2_0<=D2_des，则调用函数func2，输出期望的k1、k2_1和k2_2。同样在二区结束时，
%    应当同时实现期望航向角和期望偏移量。
% 3、若D2_0>D2_des_max，则调用函数F,2，输出期望的k1、k2_1和k2_2，其中k2_1 = k2_2。
%    在二区结束时，应当同时实现期望航向角和期望偏移量；
%


function [K1,K2_1,K2_2,D2_End,DelteSW1]= func1(Delte_Psi1,TTLC,Kw,DelteSW0,Delte_Psi2,u,D1_Ini,Delte_Psi1Ini)
%    功能：
%    已知：初始转向盘转角，TTLC，一区期望航向角变量；离开二区时的期望航向角
%    约束：1）一区结束时，在TTLC时刻实现期望的航向角变化；
%          2）二区结束时，转向盘转角为零；
%          3）二区结束时，实现期望的航向角的航向角。
%    
%    输出： 一区转向盘转角变化率K1，二区转向盘转角变化率K2_1和K2_2，二区结束时的偏移量计算值D2
%**************************************************************************
%根据公式：Delte_Psi1 = Kw*(DelteSW0*TTLC+0.5*K1*TTLC*TTLC)，求得K1。
    K1 = -2*Delte_Psi1/(Kw*TTLC*TTLC)-2*DelteSW0/TTLC;
%根据K1，TTLC和初始转向盘转角；可以计算得到进入二区时的转向盘转角初始值DelteSW1。

    DelteSW1 = DelteSW0+K1*TTLC;
    Delte_Psi = Delte_Psi1Ini+0.5*(DelteSW0+DelteSW1)*TTLC*Kw;
%利用约束2和3，可以求得K2。
    K2 = -DelteSW1*DelteSW1*Kw/(2*(Delte_Psi2-Delte_Psi));
%根据K2，DelteSW1和车速，可以计算出二区车辆的偏移量的变化量D2和二区控制时间T2。
    T1 = (DelteSW1-DelteSW0)/K1;
    T2 = (0-DelteSW1)/K2;
%     D1 = u*((1/6)*Kw*(2*DelteSW0+DelteSW1)*T1^2+Delte_Psi1*T1);
%     D2 = u*((1/3)*Kw*T2^2*DelteSW1);
    D1 = u*((1/6)*Kw*(DelteSW1+2*DelteSW0)*T1*T1+Delte_Psi1Ini*T1);
    D2 = u*((1/3)*Kw*T2*T2*DelteSW1+Delte_Psi*T2);
    D2_End = D1+D2;     
%
%**************************************************************************
%输出：
%   K1 = K1;
    K2_1 = K2;
    K2_2 = K2;
end % end of function func1

% function [K1,K2_1,K2_2,DelteSW1]= func2(Delte_Psi1,Delte_Psi2,D1_Ini,T1,...
%                                         D2_des,LDDir,DelteSW0,u,Kw)
% %    功能：
% %    已知：一区期望航向角变化量，离开二区时的期望航向角，二区结束时的期望偏移量的绝对值
% %          车辆的车道偏离的方向，初始转向盘转角，车速。
% %    约束：1）给定一区结束时的转向盘转角，实现期望的航向角变化；
% %          2）二区结束时，偏离量实现期望偏移量；
% %          3）二区结束时，实现期望的航向角的航向角；
% %          4）二区结束时，转向盘转角为零。
% %    
% %    输出： 一区转向盘转角变化率K1，二区转向盘转角变化率K2_1和K2_2，
% %           进入二区时的转向盘转角初始值DelteSW1。
% %**************************************************************************
% %   利用约束2，3和4；可以求得DelteSW1和二区转向盘转角变化率。
% Delte_D = LDDir*D2_des-D1_Ini;
% Delte_Psi = Delte_Psi2-Delte_Psi1;
% DelteSW1 = ((4/3)*(Delte_Psi/Kw)*(Delte_Psi/Kw)-(1/3)*(Delte_Psi/Kw)*DelteSW0*T1-(1/6)*DelteSW0*DelteSW0*T1*T1...
%             +2*(Delte_Psi/Kw)*Delte_Psi1-Delte_Psi1*DelteSW0*T1)/(Delte_D/(Kw*u)+(1/3)*(Delte_Psi/Kw)*T1);
% T2 = (2*(Delte_Psi/Kw)-(DelteSW1+DelteSW0)*T1)/DelteSW1;
% K2 = -DelteSW1/T2;
% %   利用约束1和进入二区时的转向盘转角初始值DelteSW1；可以求得一区转向盘转角变化率。
% K1 = (DelteSW1-DelteSW0)/T1;
% %
% %**************************************************************************
% %   输出：
% K2_1 = K2;
% K2_2 = K2;
% 
% end % end of function func1
function [T1,T2,D2_End] = func3(Delte_Psi1Ini,Delte_Psi2,DelteSW1,KMax,Delte_Psi1,...
                                DelteSW0,u,Kw,LDDir)
%    功能：
%    已知：进入一区时初始航向角，离开二区时的期望航向角，进入一区时的偏移量的初始值
%          进入二区时的转向盘转角初始值，初始转向盘转角，车速。
%    步骤：1）给定一区结束时的转向盘转角，实现一区的期望的航向角变化；
%          2）给定一区结束时的转向盘转角，实现二区的期望的航向角变化；
%          3）计算实现一区的期望的航向角变化，所产生的一区偏移量变化量D1；
%          4）计算实现二区的期望的航向角变化，所产生的二区偏移量变化量D2；
%          5) 根据进入一区时的偏移量的初始值和D1和D2，得到二区结束时的偏移量D2_End
%    
%    输出： 一区使用时间T1，二区使用时间T2，二区结束时的偏移量D2_End
%**************************************************************************
K1_0 = (DelteSW1*DelteSW1-DelteSW0*DelteSW0)*Kw/(-2*Delte_Psi1);
if (LDDir*K1_0 > KMax)
    K1_1 = single(LDDir*KMax);
else
    K1_1 = K1_0;
end
%
T1 = (DelteSW1-DelteSW0)/K1_1;

    
Delte_Psi = Delte_Psi1Ini+0.5*(DelteSW0+DelteSW1)*T1*Kw;
% DelteSW1_0 = 2*(Delte_Psi2-Delte_Psi1Ini)/(T1*Kw)-DelteSW0;
% if (-1*Delte_Psi >= -1*Delte_Psi2)
%    DelteSW1_1 = DelteSW1_0;
% else
%    DelteSW1_1 = DelteSW1;
% end
% Delte_Psi_1 = Delte_Psi1Ini+0.5*(DelteSW0+DelteSW1_1)*T1*Kw;
T2 = 2*(Delte_Psi2-Delte_Psi)/(DelteSW1*Kw);

%     T1 = 2*(Delte_Psi-Delte_Psi1)/((DelteSW0+DelteSW1)*Kw);
%     T1 = TTLC;
%     T2 = 2*(Delte_Psi2-Delte_Psi)/(DelteSW1*Kw);
    D1 = u*((1/6)*Kw*(DelteSW1+2*DelteSW0)*T1*T1+Delte_Psi1Ini*T1); 
    D2 = u*((1/3)*Kw*T2*T2*DelteSW1+Delte_Psi*T2);
    D2_End = D2+D1;
end

== matlab function LKAS_AutoSave_20200911_1102/LKAS/LL/LLOn/LKA/LKA Motion Planning (LKAMP) /Motion Planning Input Processing (MPInP)/MATLAB Function ==
  data: Actflg input; phiSWA input; phiSWA0 output; phiFf input
function phiSWA0 = fcn(Actflg, phiSWA, phiFf)
    if Actflg == 1
        phiSWA0 = min(phiSWA, phiFf);
    elseif Actflg ==2 
        phiSWA0 = max(phiSWA, phiFf);
    else
        phiSWA0 = phiSWA;
    end
end

== matlab function LKAS_AutoSave_20200911_1102/LKAS/LL/LLOn/LKA/LKA Motion Planning (LKAMP) /Steering Wheel Angle Command Calculation (SWACmdCal)/SWACmd ==
  data: SWACmd_dphi1PhSWAGrad input; SWACmd_phi2PhSWAIni input; SWACmd_dphi2PhSWAGrad input; SWACmd_phi1PhSWAIni input; SWACmd_phiSWACmd output single; SWACmd_tiNomT input; T1 output single; T2 output
 function [SWACmd_phiSWACmd,T1,T2] = SWACmd(SWACmd_dphi1PhSWAGrad,...
                                                      SWACmd_phi2PhSWAIni,...
                                                      SWACmd_dphi2PhSWAGrad,...
                                                      SWACmd_phi1PhSWAIni,...
                                                      SWACmd_tiNomT)                      
% *************************************************************************
% 输入量：
%   SWACmd_phi1PhSWAIni : 一区转向盘转角初始值，单位：deg
%   SWACmd_dphi1PhSWAGrad : 一区转向盘转角变化率，单位：deg/s
%   SWACmd_phi2PhSWAIni : 二区转向盘转角初始值，单位：deg
%   SWACmd_dphi2PhSWAGrad : 二区转向盘转角变化率，单位：deg/s
%   SWACmd_vVehSpdIni : 进入一区的车速初始值，单位：Km/h
%   SWACmd_tiNomT : 名义时间，单位：s
%
% 输出量：
%   SWACmd_phiSWACmd : 转向盘转角指令值，单位：deg
%  
%**************************************************************************
%
    DelteSW0 = SWACmd_phi1PhSWAIni; 
    DelteSW1 = SWACmd_phi2PhSWAIni;
    Delte1PhSWGrad = SWACmd_dphi1PhSWAGrad;
    Delte2PhSWGrad = SWACmd_dphi2PhSWAGrad;
    DelteSWCmd = single(0);
    NomT = SWACmd_tiNomT;
    T1 = (DelteSW1-DelteSW0)/Delte1PhSWGrad;
    T2 = (0-DelteSW1)/Delte2PhSWGrad+T1;
%**************************************************************************
%已知： 一区转向盘转角初始值， 一区转向盘转角变化率， 二区转向盘转角初始值, 
%       二区转向盘转角变化率, 进入一区的车速初始值, 行驶路径长度。
%根据车速初始值和行驶路径长度，可以计算出名义时间（NomT）；然后利用名义时间和
%方向盘运动曲线，求得转向盘转角指令值。
%
%**************************************************************************                                
if(NomT < T1 && NomT >= 0 )
    DelteSWCmd = DelteSW0+Delte1PhSWGrad*NomT;
elseif(NomT <= T2 && NomT >= T1 )
%    DelteSWCmd = DelteSW1+Delte2PhSWGrad*(NomT-T1);
    DelteSWCmd = DelteSW0+Delte1PhSWGrad*T1;
%    DelteSWCmd = single(0);
elseif(NomT >= T2)
    DelteSWCmd = DelteSW0+Delte1PhSWGrad*T1;
%   DelteSWCmd = single(0);
end
%
%**************************************************************************
% 输出：
    SWACmd_phiSWACmd = DelteSWCmd;
end

== matlab function LKAS_AutoSave_20200911_1102/LKAS/LL/LLOn/LKA/Lane Following (LF)/Trajectory Following Control (TFC)/Feedback Control (FbCtl)/Saturable Gain Lut (SatGainLut) ==
  data: Input input single [0..180]; Gain output single [10..400]; InputLimLwr input single; InputLimUpr input single; GainLimLwr input single; GainLimUpr input single
%% Function Name: Saturable Gain Lut
%
% Description: 
%   Saturable Gain Lookup Table.
%
% Assumptions and Limitation:
%   The data type of all inputs and output is single.
%
% Inputs:
%   Input:
%   InputLimLwr:
%   InputLimUpr:
%   GainLimLwr:
%   GainLimUpr:
%
% Outputs:
%   Gain: The result of Looking up table.

% $Revision: 1.0$
% $Author: Zhang Jianwei$
% $Date: January 27, 2019$
% ________________________________________
function Gain = fcn(Input, InputLimLwr, InputLimUpr, GainLimLwr, GainLimUpr)
%#eml
if Input <= InputLimLwr
    Gain = GainLimLwr;
elseif Input >= InputLimUpr
        Gain = GainLimUpr;
else Gain = (Input - InputLimLwr)/(InputLimUpr - InputLimLwr)...
        *(GainLimUpr - GainLimLwr) + GainLimLwr;
end
end

== matlab function LKAS_AutoSave_20200911_1102/LKAS/LL/LLOn/LKA Input Processing (LKAInP)/Predicted Deviation Calculation (PrDvt)/Predicted Deviation of Left Line (PrdcDvtLft)/  ==
  data: u1 input; y output; u2 input; u3 input
function y = fcn(u1,u2,u3)
y = u2*cos(u1)+u3*sin(u1);

== matlab function LKAS_AutoSave_20200911_1102/LKAS/LL/LLOn/LKA Input Processing (LKAInP)/Predicted Deviation Calculation (PrDvt)/Predicted Deviation of Left Line (PrdcDvtLft)/MATLAB Function ==
  data: u1 input; y output; u2 input
function y = fcn(u1,u2)
y = u1*cos(u2);

== matlab function LKAS_AutoSave_20200911_1102/LKAS/LL/LLOn/LKA Input Processing (LKAInP)/Predicted Deviation Calculation (PrDvt)/Predicted Deviation of Right  Line (PrdcDvtRgt)/  ==
  data: u1 input; y output; u2 input; u3 input
function y = fcn(u1,u2,u3)
y = u2*cos(u1)-u3*sin(u1);

== matlab function LKAS_AutoSave_20200911_1102/LKAS/LL/LLOn/LKA Input Processing (LKAInP)/Predicted Deviation Calculation (PrDvt)/Predicted Deviation of Right  Line (PrdcDvtRgt)/MATLAB Function ==
  data: u1 input; y output; u2 input
function y = fcn(u1,u2)
y = u1*cos(u2);

== matlab function LKAS_AutoSave_20200911_1102/LKAS/LL/LLOn/LKA Input Processing (LKAInP)/TTLC Calculation (TTLCCalc)/MATLAB Function ==
  data: dvt input; vy input; TTLC output; cur input
function TTLC = fcn(dvt, vy, cur)
    if dvt>single(0) && dvt<single(2) && vy<single(0) && vy>single(-1.5)
        TTLC = -dvt/vy;
    else
        TTLC = single(3);
    end
end

== matlab function LKAS_AutoSave_20200911_1102/LKAS/LL/LLOn/LKA Input Processing (LKAInP)/TTLC Calculation (TTLCCalc)/MATLAB Function1 ==
  data: dvt input; vy input; TTLC output; cur input
function TTLC = fcn(dvt, vy, cur)
    if dvt>single(0) && dvt<single(2) && vy<single(0) && vy>single(-1.5)
        TTLC = (-dvt)/vy;
    else
        TTLC = single(3);
    end
end

== matlab function LKAS_AutoSave_20200911_1102/LKAS/LL/LLOn/LKA Input Processing (LKAInP)/TTLC Calculation (TTLCCalc)/MATLAB Function2 ==
  data: crPrvwCrvtLft input; crPrvwCrvtRgt input; LTLC input; LFTTTLC output; RTLC input; LTTLC input; RTTLC input; RGTTTLC output; TLft input; TRgt input
function [LFTTTLC,RGTTTLC] = fcn(crPrvwCrvtLft, crPrvwCrvtRgt, LTLC, RTLC, LTTLC, RTTLC ,TLft, TRgt)
    if abs(LTTLC-LTLC)/LTTLC <= single(0.2)
        LFTTTLC = min(LTTLC,LTLC);
    else
        LFTTTLC = LTTLC;
    end
    
    if abs(RTTLC-RTLC)/RTTLC <= single(0.2)
        RGTTTLC = min(RTTLC,RTLC);
    else
        RGTTTLC = RTTLC;
    end
    
    if abs(crPrvwCrvtLft)>single(0.001) && abs(TLft-LFTTTLC)/LFTTTLC <= single(0.7) && TLft>single(0.5) && LFTTTLC <= single(1.95)
        LFTTTLC = (LFTTTLC+TLft)/single(2);
    end
    if abs(crPrvwCrvtRgt)>single(0.001) && abs(TRgt-RGTTTLC)/RGTTTLC <= single(0.7) && TRgt>single(0.5) && RGTTTLC <= single(1.95)
        RGTTTLC = (RGTTTLC+TRgt)/single(2);
    end
end

== matlab function LKAS_AutoSave_20200911_1102/LKAS/LL/LLOn/LKA Input Processing (LKAInP)/TTLC Calculation (TTLCCalc)/MATLAB Function3 ==
  data: c0 input; TLft output; c1 input; c2 input; vx input; c20 input; w input
function TLft = fcn(c0,c1,c2,vx,c20,w)
%   y1=c0+c1*x+c2*x^2+c3*x^3
%   y2=-W + C20*x^2
%   y1-y2 =(c2-c20)*x^2+c1*x+(c0+w)=0
%   b2-4ac=c1^2-4*(c2-c20)*(c0+w)
    if (c2-c20)<=single(0.001) && ((c1 > 0) || (c1 < 0))
        if (-c0-w)/c1>0
            TLft = (-c0-w)/c1/vx;
        else
            TLft = single(3);
        end
    elseif ((c2-c20)>single(0.001)) && (c1^2-4*(c2-c20)*(c0+w) >= 0)
        x10= (-c1+sqrt(c1^2-4*(c2-c20)*(c0+w)))/(2*(c2-c20));
        x20= (-c1-sqrt(c1^2-4*(c2-c20)*(c0+w)))/(2*(c2-c20));
        x1 = max(x10,x20);
        x2 = min(x10,x20);
        if x2>0
            TLft = x2/vx;
        elseif x1>0
            TLft = x1/vx;
        else
            TLft = single(3);
        end
    else
        TLft = single(3);
    end
    TLft =max(single(0.6),min(TLft,single(2)));
end

== matlab function LKAS_AutoSave_20200911_1102/LKAS/LL/LLOn/LKA Input Processing (LKAInP)/TTLC Calculation (TTLCCalc)/MATLAB Function4 ==
  data: c0 input; TRgt output; c1 input; c2 input; vx input; c20 input; w input
function TRgt = fcn(c0,c1,c2,vx,c20,w)
%   y1=c0+c1*x+c2*x^2+c3*x^3
%   y2=W + C20*x^2
%   y1-y2 =(c2-c20)*x^2+c1*x+(c0-w)=0
%   b2-4ac=c1^2-4*(c2-c20)*(c0-w)
    if (c2-c20)<=single(0.001) && ((c1 > 0) || (c1 < 0))
        if (-c0+w)/c1>0
            TRgt = (-c0+w)/c1/vx;
        else
            TRgt = single(3);
        end
    elseif ((c2-c20)>single(0.001)) && (c1^2-4*(c2-c20)*(c0-w) >= 0)
        x10= (-c1+sqrt(c1^2-4*(c2-c20)*(c0-w)))/(2*(c2-c20));
        x20= (-c1-sqrt(c1^2-4*(c2-c20)*(c0-w)))/(2*(c2-c20));
        x1 = max(x10,x20);
        x2 = min(x10,x20);
        if x2>0
            TRgt = x2/vx;
        elseif x1>0
            TRgt = x1/vx;
        else
            TRgt = single(3);
        end
    else
        TRgt = single(3);
    end
    TRgt =max(single(0.6),min(TRgt,single(2)));
end

== matlab function LKAS_AutoSave_20200911_1102/LKAS/LL/LLOn/LKA Input Processing (LKAInP)/Under The Limit (UndrLim)/Steering Wheel Angel Max (SWAMax)/MATLAB Function ==
  data: v input; SWAmax output; ax input; i input; L input; K input
function SWAmax = get_SWAmax(v,ax,i,L,K)
SWAmax = ((K*v*v+1)*ax*i*L)/(v*v)*180/3.14;

== matlab function LKAS_AutoSave_20200911_1102/LKAS/LL/LLOn/LKA Input Processing (LKAInP)/Under The Limit (UndrLim)/Steering Wheel Angel Rate Max (SWARMax)/MATLAB Function ==
  data: v input; SWARmax output; dax input; i input; L input; K input
function SWARmax = get_SWARmax(v,dax,i,L,K)
SWARmax = ((K*v*v+1)*dax*i*L)/(v*v)*180/3.14;

== stateflow chart LKAS_AutoSave_20200911_1102/LKAS/LL/LLOn/LL State Determination (LLStateDet)/LDW_State_Machine ==
  state SysOn
    state LDWSelected
      en:
      LDWSM_stLDWState = uint16(2);
    state Normal
      state LDWEnable
        en:
        LDWSM_stLDWState = uint16(3);
      state LDWLeftActive
        en:
        LDWSM_stLDWState = uint16(4);
        LDWSM_stLDWActvFlg = uint16(1);
        ex:
        LDWSM_stLDWActvFlg = uint16(0);
      state LDWRightActive
        en:
        LDWSM_stLDWState = uint16(5);
        LDWSM_stLDWActvFlg = uint16(2);
        ex:
        LDWSM_stLDWActvFlg = uint16(0);
      (default) -> LDWEnable
      LDWEnable -> LDWRightActive [order 2] : [LDWSM_stActvCSyn == 2 & LDWSM_stDeactvCSyn == 0]
      LDWEnable -> LDWLeftActive [order 1] : [LDWSM_stActvCSyn == 1 & LDWSM_stDeactvCSyn == 0]
      LDWLeftActive -> LDWEnable [order 1] : [LDWSM_stDeactvCSyn == 1]
      LDWRightActive -> LDWEnable [order 1] : [LDWSM_stDeactvCSyn == 1]
      LDWLeftActive -> LDWRightActive [order 2] : [LDWSM_stActvCSyn == 2 & LDWSM_stDeactvCSyn == 0]
      LDWRightActive -> LDWLeftActive [order 2] : [LDWSM_stActvCSyn == 1 & LDWSM_stDeactvCSyn == 0]
    (default) -> LDWSelected
    LDWSelected -> Normal : [LDWSM_stEnaCSyn == 1&LDWSM_stDisblCSyn==0]
    Normal -> LDWSelected : [LDWSM_stDisblCSyn == 1]
  state SysOff
    state Unavailable
      en:
      LDWSM_stLDWState = uint16(0);
    state Unselected
      en:
      LDWSM_stLDWState = uint16(1);
    (default) -> Unavailable
    Unavailable -> Unselected : [LDWSM_stLMCMode == 0]
  state Fault
    state LDWFault
      en:
      LDWSM_stLDWState = uint16(6);
    (default) -> LDWFault
  (default) -> SysOff
  SysOff -> SysOn [order 2] : [LDWSM_stLMCMode == 1 | LDWSM_stLMCMode == 2]
  SysOn -> Unselected [order 2] : [LDWSM_stLMCMode ~= 1 & LDWSM_stLMCMode ~= 2 ]
  Fault -> Unselected [order 2] : [LDWSM_stLMCMode == 0 & LDWSM_stFaultCSyn == 0]
  SysOff -> Fault [order 1] : [(LDWSM_stLMCMode == 1 | LDWSM_stLMCMode == 2) & LDWSM_stFaultCSyn == 1]
  SysOn -> Fault [order 1] : [LDWSM_stFaultCSyn == 1]
  Fault -> SysOn [order 1] : [LDWSM_stFaultCSyn == 0 & (LDWSM_stLMCMode == 1 | LDWSM_stLMCMode == 2) ]
  data: LDWSM_stLDWActvFlg output uint8 [0..7]; LDWSM_stLDWState output uint8 [0..7]; LDWSM_stLMCMode input uint8 [0..5]; LDWSM_stEnaCSyn input boolean [0..1]; LDWSM_stDisblCSyn input boolean [0..1]; LDWSM_stActvCSyn input uint8 [0..3]; LDWSM_stDeactvCSyn input boolean [0..1]; LDWSM_stFaultCSyn input boolean [0..1]
  data LDWSM_stLDWActvFlg settings: description=|
      | 0 -- Deactive
      | 1 -- Left Active
      | 2 -- Right Active
  data LDWSM_stLDWState settings: description=|
      | 0 -- Unavailable
      | 1 -- Unselected
      | 2 -- Selected
      | 3 -- Enabled
      | 4 -- Left Active
      | 5 -- Right Active
      | 6 -- Fault
      | 7 -- Reserved
  data LDWSM_stLMCMode settings: description=|
      | 0 -- Unselected
      | 1 -- LDWMode
      | 2 -- LKAMode
      | 3 -- TJAMode
      | 4 -- HWAMode
      | 5 -- Reserved
  data LDWSM_stEnaCSyn settings: description=|
      | 0 -- No Enable
      | 1 -- LDW Enable
      | 2 -- LKA Enable
      | 3 -- Reserved
  data LDWSM_stDisblCSyn settings: description=|
      | 0 -- No Disable
      | 1 -- LDW Disable
      | 2 -- LKA Disable
      | 3 -- Reserved
  data LDWSM_stActvCSyn settings: description=|
      | 0 -- No Active
      | 1 -- LDW Left Active
      | 2 -- LDW Right Active
      | 3 -- LKA Left Active
      | 4 -- LKA Right Active
      | 5 -- Reserved
  data LDWSM_stDeactvCSyn settings: description=|
      | 0 -- No Deactive
      | 1 -- LDW Deactive
      | 2 -- LKA Deactive
      | 3 -- Reserved
  data LDWSM_stFaultCSyn settings: description=|
      | 0 -- No Fault
      | 1 -- LDW Fault
      | 2 -- LKA Fault
      | 3 -- Reserved

== stateflow chart LKAS_AutoSave_20200911_1102/LKAS/LL/LLOn/LL State Determination (LLStateDet)/LKA_State_Machine ==
  state SysOn
    state LKASelected
      en:
      LKASM_stLKAState = uint16(2);
    state Normal
      state LKAEnable
        en:
        LKASM_stLKAState = uint16(3);
      state LKALeftActive
        en:
        LKASM_stLKAState = uint16(4);
        LKASM_stLKAActvFlg = uint16(1);
        ex:
        LKASM_stLKAActvFlg = uint16(0);
      state LKARightActive
        en:
        LKASM_stLKAState = uint16(5);
        LKASM_stLKAActvFlg = uint16(2);
        ex:
        LKASM_stLKAActvFlg = uint16(0);
      (default) -> LKAEnable
      LKAEnable -> LKARightActive [order 2] : [LKASM_stActvCSyn == 2 & LKASM_stDeactvCSyn ==0 ]
      LKAEnable -> LKALeftActive [order 1] : [LKASM_stActvCSyn == 1 & LKASM_stDeactvCSyn ==0 ]
      LKALeftActive -> LKAEnable [order 1] : [LKASM_stDeactvCSyn ==1 ]
      LKARightActive -> LKAEnable [order 1] : [LKASM_stDeactvCSyn == 1]
      LKALeftActive -> LKARightActive [order 2] : [LKASM_stActvCSyn == 2 & LKASM_stDeactvCSyn ==0]
      LKARightActive -> LKALeftActive [order 2] : [LKASM_stActvCSyn == 1 & LKASM_stDeactvCSyn ==0]
    (default) -> LKASelected
    LKASelected -> Normal : [LKASM_stEnaCSyn == 1&LKASM_stDisblCSyn ==0]
    Normal -> LKASelected : [LKASM_stDisblCSyn ==1]
  state SysOff
    state Unavailable
      en:
      LKASM_stLKAState = uint16(0);
    state Unselected
      en:
      LKASM_stLKAState = uint16(1);
    (default) -> Unavailable
    Unavailable -> Unselected : [LKASM_stLMCMode == 0 | LKASM_stLMCMode == 1]
  state Fault
    state LKAFault
      en:
      LKASM_stLKAState = uint16(6);
    (default) -> LKAFault
  (default) -> SysOff
  SysOff -> SysOn [order 2] : [LKASM_stLMCMode == 2]
  SysOn -> Unselected [order 2] : [LKASM_stLMCMode ~= 2]
  Fault -> Unselected [order 2] : [(LKASM_stLMCMode == 0 | LKASM_stLMCMode == 1) & LKASM_stFaultCSyn == 0]
  SysOff -> Fault [order 1] : [LKASM_stLMCMode == 2 & LKASM_stFaultCSyn == 1 ]
  SysOn -> Fault [order 1] : [LKASM_stFaultCSyn == 1 ]
  Fault -> SysOn [order 1] : [LKASM_stFaultCSyn == 0 & LKASM_stLMCMode == 2]
  data: LKASM_stLKAActvFlg output uint8 [0..7]; LKASM_stLKAState output uint8 [0..7]; LKASM_stLMCMode input uint8 [0..5]; LKASM_stEnaCSyn input boolean [0..1]; LKASM_stDisblCSyn input boolean [0..1]; LKASM_stActvCSyn input uint8 [0..3]; LKASM_stDeactvCSyn input boolean [0..1]; LKASM_stFaultCSyn input boolean [0..1]
  data LKASM_stLKAActvFlg settings: description=|
      | 0 -- Deactive
      | 1 -- Left Active
      | 2 -- Right Active
  data LKASM_stLKAState settings: description=|
      | 0 -- Unavailable
      | 1 -- Unselected
      | 2 -- Selected
      | 3 -- Enabled
      | 4 -- Left Active
      | 5 -- Right Active
      | 6 -- Fault
      | 7 -- Reserved
  data LKASM_stLMCMode settings: description=|
      | 0 -- Unselected
      | 1 -- LDWMode
      | 2 -- LKAMode
      | 3 -- TJAMode
      | 4 -- HWAMode
      | 5 -- Reserved
  data LKASM_stEnaCSyn settings: description=|
      | 0 -- No Enable
      | 1 -- LDW Enable
      | 2 -- LKA Enable
      | 3 -- Reserved
  data LKASM_stDisblCSyn settings: description=|
      | 0 -- No Disable
      | 1 -- LDW Disable
      | 2 -- LKA Disable
      | 3 -- Reserved
  data LKASM_stActvCSyn settings: description=|
      | 0 -- No Active
      | 1 -- LDW Left Active
      | 2 -- LDW Right Active
      | 3 -- LKA Left Active
      | 4 -- LKA Right Active
      | 5 -- Reserved
  data LKASM_stDeactvCSyn settings: description=|
      | 0 -- No Deactive
      | 1 -- LDW Deactive
      | 2 -- LKA Deactive
      | 3 -- Reserved
  data LKASM_stFaultCSyn settings: description=|
      | 0 -- No Fault
      | 1 -- LDW Fault
      | 2 -- LKA Fault
      | 3 -- Reserved

== matlab function LKAS_AutoSave_20200911_1102/LKAS/LL/LLOn/LL State Determination (LLStateDet)/LL State Machine Conditions (LLSMCon)/Deactivation Condition (DeactvC)/Driver Take Condition (DvrTkCon)/MATLAB Function ==
  data: stActvFlg input; stDvrTkConFlg output; EPSTrq input; VehSpd input; DisableTrq input; CrvtTrq input
function stDvrTkConFlg = fcn(stActvFlg, EPSTrq, VehSpd, DisableTrq, CrvtTrq)
    Spd = single(min(max(single(60),VehSpd),single(80)));
    MidTqlmt = single((single(1.5)*DisableTrq-Spd/single(120)*DisableTrq)*single(0.8) + CrvtTrq);
    if stActvFlg == 2 && EPSTrq > MidTqlmt
        stDvrTkConFlg=1;
    elseif stActvFlg == 1 && EPSTrq < single(-1)*MidTqlmt
        stDvrTkConFlg=1;
    else
        stDvrTkConFlg=0;
    end
end

== matlab function LKAS_AutoSave_20200911_1102/LKAS/LL/LLOn/LL State Determination (LLStateDet)/LL State Machine Conditions (LLSMCon)/Disable Condition (DisblC)/Subsystem/C1 ==
  data: u input; y output
function y = fcn(u)
if u==0

  y=1;
else
    y=0;
end

== matlab function LKAS_AutoSave_20200911_1102/LKAS/LL/LLOn/LL State Determination (LLStateDet)/LL State Machine Conditions (LLSMCon)/Disable Condition (DisblC)/Subsystem/CURVAT ==
  data: u input; y output
function y = fcn(u)
if u==0

  y=1;
else
    y=0;
end

== matlab function LKAS_AutoSave_20200911_1102/LKAS/LL/LLOn/LL State Determination (LLStateDet)/LL State Machine Conditions (LLSMCon)/Disable Condition (DisblC)/Subsystem/GEAR ==
  data: u input; y output
function y = fcn(u)
if u==0

  y=1;
else
    y=0;
end

== matlab function LKAS_AutoSave_20200911_1102/LKAS/LL/LLOn/LL State Determination (LLStateDet)/LL State Machine Conditions (LLSMCon)/Disable Condition (DisblC)/Subsystem/LDWOwn ==
  data: u input; y output
function y = fcn(u)
if u==0

  y=1;
else
    y=0;
end

== matlab function LKAS_AutoSave_20200911_1102/LKAS/LL/LLOn/LL State Determination (LLStateDet)/LL State Machine Conditions (LLSMCon)/Disable Condition (DisblC)/Subsystem/LDWTimeOut ==
  data: u input; y output
function y = fcn(u)
if u==0

  y=1;
else
    y=0;
end

== matlab function LKAS_AutoSave_20200911_1102/LKAS/LL/LLOn/LL State Determination (LLStateDet)/LL State Machine Conditions (LLSMCon)/Disable Condition (DisblC)/Subsystem/LIGHT ==
  data: u input; y output
function y = fcn(u)
if u==0

  y=1;
else
    y=0;
end

== matlab function LKAS_AutoSave_20200911_1102/LKAS/LL/LLOn/LL State Determination (LLStateDet)/LL State Machine Conditions (LLSMCon)/Disable Condition (DisblC)/Subsystem/LKA_EPS ==
  data: u input; y output
function y = fcn(u)
if u==0

  y=1;
else
    y=0;
end
